simulink model "fullstate_sim"  (R2020a)
settings: Solver=VariableStepAuto  StartTime=0.0  StopTime=5  RelTol=1e-6
undefined symbols (not defined in the file): A, B, C_full, D_full, icd, K
settings Model: Creator=Jasper  LastModifiedBy=Jasper

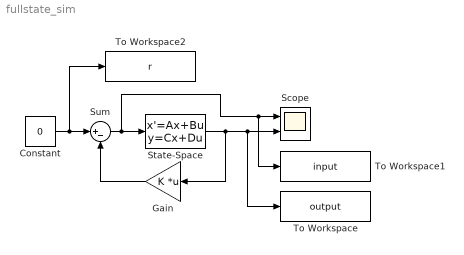
== system fullstate_sim ==
  Constant : Constant  Value=0
  Gain : Gain  Gain=K  Multiplication=Matrix(K*u)
  Scope : Scope  NumInputPorts=2
  State-Space : StateSpace  A=A  B=B  C=C_full  D=D_full  InitialCondition=icd
  Sum : Sum  Inputs=|+-
  To Workspace : ToWorkspace  VariableName=output  SaveFormat=Timeseries  SampleTime=-1
  To Workspace1 : ToWorkspace  VariableName=input  SaveFormat=Timeseries  SampleTime=-1
  To Workspace2 : ToWorkspace  VariableName=r  SaveFormat=Timeseries  SampleTime=-1
  wires:
  State-Space/1 -> To Workspace/1, Scope/2, Gain/1
  Gain/1 -> Sum/2
  Sum/1 -> To Workspace1/1, Scope/1, State-Space/1
  Constant/1 -> To Workspace2/1, Sum/1
